simulink model "Approx_Multiplier_M2_AMA2_NAB12"  (R2021a)
settings: Solver=VariableStepAuto  StartTime=0.0  StopTime=0.01  RelTol=1e-3
(part 1 of 2)
settings Model: SimulationMode=accelerator  Creator=PC  LastModifiedBy=PC
settings DataIOCC: SaveOutput=off  SignalLogging=off  DSMLogging=off  SaveTime=off

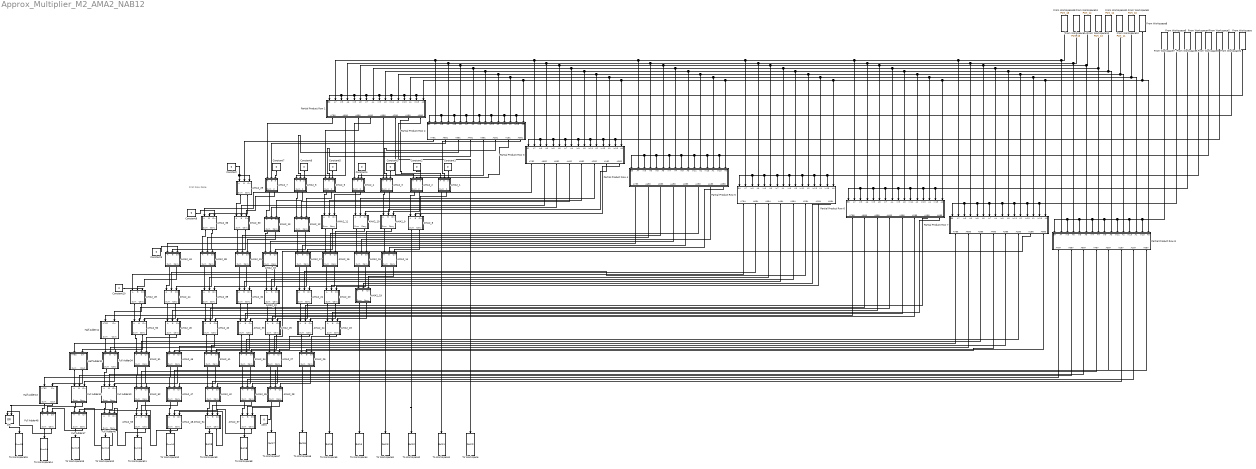
== system Approx_Multiplier_M2_AMA2_NAB12 ==
  note: First Row Done
  AMA2_1 : Subsystem
  AMA2_10 : Subsystem
  AMA2_11 : Subsystem
  AMA2_12 : Subsystem
  AMA2_13 : Subsystem
  AMA2_14 : Subsystem
  AMA2_15 : Subsystem
  AMA2_16 : Subsystem
  AMA2_17 : Subsystem
  AMA2_18 : Subsystem
  AMA2_19 : Subsystem
  AMA2_2 : Subsystem
  AMA2_20 : Subsystem
  AMA2_21 : Subsystem
  AMA2_22 : Subsystem
  AMA2_23 : Subsystem
  AMA2_24 : Subsystem
  AMA2_25 : Subsystem
  AMA2_26 : Subsystem
  AMA2_27 : Subsystem
  AMA2_28 : Subsystem
  AMA2_29 : Subsystem
  AMA2_3 : Subsystem
  AMA2_30 : Subsystem
  AMA2_31 : Subsystem
  AMA2_32 : Subsystem
  AMA2_33 : Subsystem
  AMA2_34 : Subsystem
  AMA2_35 : Subsystem
  AMA2_36 : Subsystem
  AMA2_37 : Subsystem
  AMA2_38 : Subsystem
  AMA2_39 : Subsystem
  AMA2_4 : Subsystem
  AMA2_40 : Subsystem
  AMA2_41 : Subsystem
  AMA2_42 : Subsystem
  AMA2_43 : Subsystem
  AMA2_44 : Subsystem
  AMA2_45 : Subsystem
  AMA2_46 : Subsystem
  AMA2_47 : Subsystem
  AMA2_48 : Subsystem
  AMA2_49 : Subsystem
  AMA2_5 : Subsystem
  AMA2_50 : Subsystem
  AMA2_51 : Subsystem
  AMA2_52 : Subsystem
  AMA2_53 : Subsystem
  AMA2_54 : Subsystem
  AMA2_6 : Subsystem
  AMA2_7 : Subsystem
  AMA2_8 : Subsystem
  AMA2_9 : Subsystem
  Constant{,1..10} (11 alike) : Constant  Value=0
  From Workspace : FromWorkspace  VariableName=Port_1
  From Workspace1 : FromWorkspace  VariableName=Port_2
  From Workspace10 : FromWorkspace  VariableName=Port_11
  From Workspace11 : FromWorkspace  VariableName=Port_12
  From Workspace12 : FromWorkspace  VariableName=Port_13
  From Workspace13 : FromWorkspace  VariableName=Port_14
  From Workspace14 : FromWorkspace  VariableName=Port_15
  From Workspace15 : FromWorkspace  VariableName=Port_16
  From Workspace2 : FromWorkspace  VariableName=Port_3
  From Workspace3 : FromWorkspace  VariableName=Port_4
  From Workspace4 : FromWorkspace  VariableName=Port_5
  From Workspace5 : FromWorkspace  VariableName=Port_6
  From Workspace6 : FromWorkspace  VariableName=Port_7
  From Workspace7 : FromWorkspace  VariableName=Port_8
  From Workspace8 : FromWorkspace  VariableName=Port_9
  From Workspace9 : FromWorkspace  VariableName=Port_10
  Full Adder34 : Subsystem
  Full Adder40 : Subsystem
  Full Adder41 : Subsystem
  Full Adder46 : Subsystem
  Full Adder47 : Subsystem
  Full Adder48 : Subsystem
  Half Adder11 : Subsystem
  Half Adder12 : Subsystem
  Half Adder13 : Subsystem
  OR : Logic  Operator=OR  IconShape=distinctive  AllPortsSameDT=off  OutDataTypeStr=boolean
  Partial Product Row 1 : Subsystem
  Partial Product Row 2 : Subsystem
  Partial Product Row 3 : Subsystem
  Partial Product Row 4 : Subsystem
  Partial Product Row 5 : Subsystem
  Partial Product Row 6 : Subsystem
  Partial Product Row 7 : Subsystem
  Partial Product Row 8 : Subsystem
  To Workspace : ToWorkspace  VariableName=Sum0  SampleTime=0.01
      settings: Save2DSignal=2-D array (concatenate along first dimension)
  To Workspace1 : ToWorkspace  VariableName=Sum1  SampleTime=0.01
      settings: Save2DSignal=2-D array (concatenate along first dimension)
  To Workspace10 : ToWorkspace  VariableName=Sum10  SampleTime=0.01
      settings: Save2DSignal=2-D array (concatenate along first dimension)
  To Workspace11 : ToWorkspace  VariableName=Sum11  SampleTime=0.01
      settings: Save2DSignal=2-D array (concatenate along first dimension)
  To Workspace12 : ToWorkspace  VariableName=Sum12  SampleTime=0.01
      settings: Save2DSignal=2-D array (concatenate along first dimension)
  To Workspace13 : ToWorkspace  VariableName=Sum13  SampleTime=0.01
      settings: Save2DSignal=2-D array (concatenate along first dimension)
  To Workspace14 : ToWorkspace  VariableName=Sum14  SampleTime=0.01
      settings: Save2DSignal=2-D array (concatenate along first dimension)
  To Workspace15 : ToWorkspace  VariableName=Sum15  SampleTime=0.01
      settings: Save2DSignal=2-D array (concatenate along first dimension)
  To Workspace2 : ToWorkspace  VariableName=Sum2  SampleTime=0.01
      settings: Save2DSignal=2-D array (concatenate along first dimension)
  To Workspace3 : ToWorkspace  VariableName=Sum3  SampleTime=0.01
      settings: Save2DSignal=2-D array (concatenate along first dimension)
  To Workspace4 : ToWorkspace  VariableName=Sum4  SampleTime=0.01
      settings: Save2DSignal=2-D array (concatenate along first dimension)
  To Workspace5 : ToWorkspace  VariableName=Sum5  SampleTime=0.01
      settings: Save2DSignal=2-D array (concatenate along first dimension)
  To Workspace6 : ToWorkspace  VariableName=Sum6  SampleTime=0.01
      settings: Save2DSignal=2-D array (concatenate along first dimension)
  To Workspace7 : ToWorkspace  VariableName=Sum7  SampleTime=0.01
      settings: Save2DSignal=2-D array (concatenate along first dimension)
  To Workspace8 : ToWorkspace  VariableName=Sum8  SampleTime=0.01
      settings: Save2DSignal=2-D array (concatenate along first dimension)
  To Workspace9 : ToWorkspace  VariableName=Sum9  SampleTime=0.01
      settings: Save2DSignal=2-D array (concatenate along first dimension)
  Zero : Constant  Value=0  OutDataTypeStr=Inherit: Inherit via back propagation
  wires:
  Partial Product Row 5/7(A1B4) -> AMA2_20/2(B)
  AMA2_9/2(Carry) -> AMA2_15/3(Cin)
  Partial Product Row 8/7(A1B7) -> AMA2_35/2(B)
  Full Adder48/1(Sum) -> To Workspace14/1
  Partial Product Row 4/7(A1B3) -> AMA2_15/2(B)
  Half Adder11/2(Cout) -> Half Adder12/2(Cin)
  AMA2_8/2(Carry) -> AMA2_14/3(Cin)
  Partial Product Row 6/8(A0B5) -> AMA2_23/2(B)
  AMA2_10/1(Sum) -> AMA2_15/1(A)
  From Workspace14/1 -> Partial Product Row 8/4(A6), Partial Product Row 7/4(A6), Partial Product Row 6/4(A6), Partial Product Row 5/4(A6), Partial Product Row 4/4(A6), Partial Product Row 3/4(A6), Partial Product Row 1/4(A6), Partial Product Row 2/4(A6)
  AMA2_12/1(Sum) -> AMA2_17/1(A)
  AMA2_43/2(Carry) -> AMA2_49/2(B)
  AMA2_24/2(Carry) -> AMA2_27/3(Cin)
  Partial Product Row 7/2(A6B6) -> Full Adder34/2(B)
  Partial Product Row 1/6(A2B0) -> AMA2_2/1(A)
  Partial Product Row 2/5(A3B1) -> AMA2_4/2(B)
  Constant7/1 -> AMA2_7/3(Cin)
  AMA2_17/2(Carry) -> AMA2_22/3(Cin)
  Constant2/1 -> AMA2_2/3(Cin)
  AMA2_49/2(Carry) -> Half Adder11/2(Cin)
  AMA2_3/2(Carry) -> AMA2_10/3(Cin)
  From Workspace13/1 -> Partial Product Row 8/6(A5), Partial Product Row 6/6(A5), Partial Product Row 3/6(A5), Partial Product Row 1/6(A5), Partial Product Row 2/6(A5), Partial Product Row 4/6(A5), Partial Product Row 5/6(A5), Partial Product Row 7/6(A5)
  AMA2_12/2(Carry) -> AMA2_18/3(Cin)
  AMA2_45/2(Carry) -> AMA2_51/3(Cin)
  From Workspace8/1 -> Partial Product Row 8/16(A0), Partial Product Row 7/16(A0), Partial Product Row 6/16(A0), Partial Product Row 4/16(A0), Partial Product Row 3/16(A0), Partial Product Row 1/16(A0), Partial Product Row 2/16(A0), Partial Product Row 5/16(A0)
  Partial Product Row 1/5(A3B0) -> AMA2_3/1(A)
  Full Adder34/2(Carry) -> Full Adder41/3(Cin)
  AMA2_27/2(Carry) -> AMA2_35/3(Cin)
  AMA2_54/1(Sum) -> To Workspace9/1
  Partial Product Row 3/4(A4B2) -> AMA2_12/2(B)
  AMA2_5/2(Carry) -> AMA2_12/3(Cin)
  AMA2_6/1(Sum) -> AMA2_12/1(A)
  AMA2_13/1(Sum) -> AMA2_18/1(A)
  AMA2_2/1(Sum) -> AMA2_8/1(A)
  AMA2_11/2(Carry) -> AMA2_17/3(Cin)
  AMA2_53/1(Sum) -> To Workspace11/1
  Full Adder46/1(Sum) -> To Workspace12/1
  AMA2_34/1(Sum) -> AMA2_35/1(A)
  Partial Product Row 2/8(A0B1) -> AMA2_1/2(B)
  AMA2_8/1(Sum) -> To Workspace2/1
  Partial Product Row 3/2(A6B2) -> AMA2_30/2(B)
  AMA2_2/2(Carry) -> AMA2_9/3(Cin)
  AMA2_40/2(Carry) -> AMA2_46/3(Cin)
  AMA2_37/1(Sum) -> To Workspace8/1
  AMA2_25/1(Sum) -> AMA2_27/1(A)
  Half Adder13/1(Sum) -> Full Adder48/1(A)
  Constant3/1 -> AMA2_3/3(Cin)
  Partial Product Row 7/6(A2B6) -> AMA2_34/2(B)
  Constant4/1 -> AMA2_4/3(Cin)
  AMA2_33/1(Sum) -> AMA2_34/1(A)
  Partial Product Row 4/5(A3B3) -> AMA2_17/2(B)
  AMA2_41/2(Carry) -> AMA2_47/3(Cin)
  AMA2_18/2(Carry) -> AMA2_32/3(Cin)
  AMA2_18/1(Sum) -> AMA2_22/1(A)
  Partial Product Row 3/8(A0B2) -> AMA2_8/2(B)
  Partial Product Row 2/4(A4B1) -> AMA2_5/2(B)
  Full Adder47/2(Carry) -> Full Adder48/3(Cin)
  Partial Product Row 2/3(A5B1) -> AMA2_6/2(B)
  AMA2_53/2(Carry) -> Full Adder46/3(Cin)
  Partial Product Row 6/7(A1B5) -> AMA2_24/2(B)
  From Workspace/1 -> Partial Product Row 1/3(In3), Partial Product Row 1/1(B0), Partial Product Row 1/5(In5), Partial Product Row 1/7(In7), Partial Product Row 1/9(In9), Partial Product Row 1/11(In11), Partial Product Row 1/13(In13), Partial Product Row 1/15(In15)
  AMA2_13/2(Carry) -> AMA2_31/3(Cin)
  Partial Product Row 6/4(A4B5) -> AMA2_40/2(B)
  From Workspace12/1 -> Partial Product Row 8/8(A4), Partial Product Row 6/8(A4), Partial Product Row 4/8(A4), Partial Product Row 3/8(A4), Partial Product Row 1/8(A4), Partial Product Row 2/8(A4), Partial Product Row 5/8(A4), Partial Product Row 7/8(A4)
  AMA2_37/2(Carry) -> AMA2_54/3(Cin)
  AMA2_43/1(Sum) -> AMA2_44/1(A)
  Partial Product Row 1/7(A1B0) -> AMA2_1/1(A)
  Partial Product Row 5/6(A2B4) -> AMA2_21/2(B)
  AMA2_14/1(Sum) -> To Workspace3/1
  Partial Product Row 8/8(A0B7) -> AMA2_28/2(B)
  From Workspace5/1 -> Partial Product Row 6/7(In7), Partial Product Row 6/5(In5), Partial Product Row 6/1(B5), Partial Product Row 6/3(In3), Partial Product Row 6/9(In9), Partial Product Row 6/11(In11), Partial Product Row 6/13(In13), Partial Product Row 6/15(In15)
  Partial Product Row 1/2(A6B0) -> AMA2_6/1(A)
  AMA2_44/1(Sum) -> AMA2_45/1(A)
  AMA2_45/1(Sum) -> AMA2_46/1(A)
  AMA2_19/2(Carry) -> AMA2_23/3(Cin)
  AMA2_35/1(Sum) -> AMA2_37/1(A)
  AMA2_22/1(Sum) -> AMA2_25/1(A)
  AMA2_51/2(Carry) -> Full Adder40/3(Cin)
  AMA2_54/2(Carry) -> AMA2_48/3(Cin)
  AMA2_23/1(Sum) -> To Workspace5/1
  AMA2_48/2(Carry) -> AMA2_53/3(Cin)
  AMA2_30/2(Carry) -> AMA2_38/3(Cin)
  Partial Product Row 5/1(A7B4) -> AMA2_49/1(A)
  Constant/1 -> AMA2_29/3(Cin), AMA2_29/1(A)
  Partial Product Row 1/1(A7B0) -> AMA2_7/1(A)
  AMA2_30/1(Sum) -> AMA2_31/1(A)
  Full Adder46/2(Carry) -> Full Adder47/3(Cin)
  AMA2_31/2(Carry) -> AMA2_39/3(Cin)
  Partial Product Row 7/4(A4B6) -> AMA2_46/2(B)
  Full Adder40/1(Sum) -> Full Adder46/1(A)
  AMA2_22/2(Carry) -> AMA2_33/3(Cin)
  Partial Product Row 4/3(A5B3) -> AMA2_31/2(B)
  AMA2_20/1(Sum) -> AMA2_23/1(A)
  AMA2_42/1(Sum) -> AMA2_54/1(A)
  AMA2_15/2(Carry) -> AMA2_20/3(Cin)
  AMA2_49/1(Sum) -> AMA2_50/1(A)
  From Workspace4/1 -> Partial Product Row 5/15(In15), Partial Product Row 5/13(In13), Partial Product Row 5/11(In11), Partial Product Row 5/7(In7), Partial Product Row 5/5(In5), Partial Product Row 5/1(B4), Partial Product Row 5/3(In3), Partial Product Row 5/9(In9)
  AMA2_7/2(Carry) -> AMA2_30/3(Cin)
  From Workspace7/1 -> Partial Product Row 8/11(In11), Partial Product Row 8/9(In9), Partial Product Row 8/7(In7), Partial Product Row 8/5(In5), Partial Product Row 8/3(In3), Partial Product Row 8/1(B7), Partial Product Row 8/13(In13), Partial Product Row 8/15(In15)
  AMA2_52/1(Sum) -> AMA2_53/1(A)
  AMA2_40/1(Sum) -> AMA2_41/1(A)
  AMA2_46/1(Sum) -> AMA2_47/1(A)
  AMA2_31/1(Sum) -> AMA2_32/1(A)
  Partial Product Row 5/5(A3B4) -> AMA2_22/2(B)
  AMA2_51/1(Sum) -> AMA2_52/1(A)
  Partial Product Row 7/7(A1B6) -> AMA2_27/2(B)
  Partial Product Row 7/1(A7B6) -> Half Adder12/1(A7B2)
  AMA2_29/2(Carry) -> AMA2_36/2(B)
  AMA2_41/1(Sum) -> AMA2_42/1(A)
  AMA2_9/1(Sum) -> AMA2_14/1(A)
  AMA2_38/2(Carry) -> AMA2_44/3(Cin)
  AMA2_32/1(Sum) -> AMA2_33/1(A)
  Partial Product Row 3/6(A2B2) -> AMA2_10/2(B)
  Partial Product Row 8/1(A7B7) -> Half Adder13/1(A7B2)
  Constant1/1 -> AMA2_1/3(Cin)
  Partial Product Row 7/3(A5B6) -> AMA2_51/2(B)
  Partial Product Row 5/3(A5B4) -> AMA2_39/2(B)
  AMA2_46/2(Carry) -> AMA2_52/3(Cin)
  AMA2_29/1(Sum) -> AMA2_30/1(A)
  From Workspace6/1 -> Partial Product Row 7/13(In13), Partial Product Row 7/7(In7), Partial Product Row 7/5(In5), Partial Product Row 7/1(B6), Partial Product Row 7/3(In3), Partial Product Row 7/9(In9), Partial Product Row 7/11(In11), Partial Product Row 7/15(In15)
  Partial Product Row 2/1(A7B1) -> AMA2_29/2(B)
  From Workspace3/1 -> Partial Product Row 4/13(In13), Partial Product Row 4/11(In11), Partial Product Row 4/9(In9), Partial Product Row 4/5(In5), Partial Product Row 4/3(In3), Partial Product Row 4/1(B3), Partial Product Row 4/7(In7), Partial Product Row 4/15(In15)
  From Workspace9/1 -> Partial Product Row 8/14(A1), Partial Product Row 7/14(A1), Partial Product Row 4/14(A1), Partial Product Row 1/14(A1), Partial Product Row 2/14(A1), Partial Product Row 3/14(A1), Partial Product Row 5/14(A1), Partial Product Row 6/14(A1)
  Half Adder11/1(Sum) -> Full Adder34/1(A)
  AMA2_25/2(Carry) -> AMA2_34/3(Cin)
  AMA2_3/1(Sum) -> AMA2_9/1(A)
  AMA2_39/1(Sum) -> AMA2_40/1(A)
  Partial Product Row 7/5(A3B6) -> AMA2_41/2(B)
  Half Adder12/2(Cout) -> Half Adder13/2(Cin)
  AMA2_1/1(Sum) -> To Workspace1/1
  Partial Product Row 4/2(A6B3) -> AMA2_38/2(B)
  Partial Product Row 5/8(A0B4) -> AMA2_19/2(B)
  AMA2_10/2(Carry) -> AMA2_16/3(Cin)
  AMA2_4/2(Carry) -> AMA2_11/3(Cin)
  AMA2_17/1(Sum) -> AMA2_21/1(A)
  Partial Product Row 1/3(A5B0) -> AMA2_5/1(A)
  From Workspace15/1 -> Partial Product Row 7/2(A7), Partial Product Row 5/2(A7), Partial Product Row 3/2(A7), Partial Product Row 1/2(A7), Partial Product Row 2/2(A7), Partial Product Row 4/2(A7), Partial Product Row 6/2(A7), Partial Product Row 8/2(A7)
  AMA2_11/1(Sum) -> AMA2_16/1(A)
  Partial Product Row 6/5(A3B5) -> AMA2_33/2(B)
  Partial Product Row 2/6(A2B1) -> AMA2_3/2(B)
  AMA2_26/2(Carry) -> AMA2_28/3(Cin)
  AMA2_36/1(Sum) -> AMA2_38/1(A)
  Partial Product Row 8/5(A3B7) -> AMA2_47/2(B)
  Full Adder34/1(Sum) -> Full Adder40/1(A)
  Partial Product Row 5/2(A6B4) -> AMA2_44/2(B)
  Partial Product Row 3/3(A5B2) -> AMA2_13/2(B)
  From Workspace11/1 -> Partial Product Row 8/10(A3), Partial Product Row 6/10(A3), Partial Product Row 4/10(A3), Partial Product Row 3/10(A3), Partial Product Row 1/10(A3), Partial Product Row 2/10(A3), Partial Product Row 5/10(A3), Partial Product Row 7/10(A3)
  AMA2_50/2(Carry) -> Full Adder34/3(Cin)
  Partial Product Row 6/3(A5B5) -> AMA2_45/2(B)
  AMA2_28/1(Sum) -> To Workspace7/1
  AMA2_16/1(Sum) -> AMA2_20/1(A)
  Partial Product Row 6/2(A6B5) -> AMA2_50/2(B)
  From Workspace1/1 -> Partial Product Row 2/15(In15), Partial Product Row 2/5(In5), Partial Product Row 2/3(In3), Partial Product Row 2/1(B1), Partial Product Row 2/7(In7), Partial Product Row 2/9(In9), Partial Product Row 2/11(In11), Partial Product Row 2/13(In13)
  AMA2_26/1(Sum) -> To Workspace6/1
  From Workspace10/1 -> Partial Product Row 8/12(A2), Partial Product Row 7/12(A2), Partial Product Row 5/12(A2), Partial Product Row 4/12(A2), Partial Product Row 3/12(A2), Partial Product Row 1/12(A2), Partial Product Row 2/12(A2), Partial Product Row 6/12(A2)
  Partial Product Row 8/2(A6B7) -> Full Adder41/2(B)
  Constant5/1 -> AMA2_5/3(Cin)
  AMA2_21/2(Carry) -> AMA2_25/3(Cin)
  Partial Product Row 6/1(A7B5) -> Half Adder11/1(A7B2)
  From Workspace2/1 -> Partial Product Row 3/13(In13), Partial Product Row 3/7(In7), Partial Product Row 3/5(In5), Partial Product Row 3/3(In3), Partial Product Row 3/1(B2), Partial Product Row 3/9(In9), Partial Product Row 3/11(In11), Partial Product Row 3/15(In15)
  AMA2_48/1(Sum) -> To Workspace10/1
  AMA2_15/1(Sum) -> AMA2_19/1(A)
  AMA2_20/2(Carry) -> AMA2_24/3(Cin)
  AMA2_27/1(Sum) -> AMA2_28/1(A)
  AMA2_19/1(Sum) -> To Workspace4/1
  Partial Product Row 2/2(A6B1) -> AMA2_7/2(B)
  AMA2_14/2(Carry) -> AMA2_19/3(Cin)
  Partial Product Row 4/1(A7B3) -> AMA2_43/1(A)
  Partial Product Row 3/5(A3B2) -> AMA2_11/2(B)
  AMA2_47/1(Sum) -> AMA2_48/1(A)
  Partial Product Row 3/1(A7B2) -> AMA2_36/1(A)
  Full Adder41/1(Sum) -> Full Adder47/1(A)
  AMA2_38/1(Sum) -> AMA2_39/1(A)
  AMA2_36/2(Carry) -> AMA2_43/2(B)
  AMA2_39/2(Carry) -> AMA2_45/3(Cin)
  Partial Product Row 3/7(A1B2) -> AMA2_9/2(B)
  AMA2_32/2(Carry) -> AMA2_40/3(Cin)
  Partial Product Row 8/6(A2B7) -> AMA2_42/2(B)
  AMA2_23/2(Carry) -> AMA2_26/3(Cin)
  AMA2_5/1(Sum) -> AMA2_11/1(A)
  Partial Product Row 8/3(A5B7) -> Full Adder40/2(B)
  AMA2_6/2(Carry) -> AMA2_13/3(Cin)
  AMA2_16/2(Carry) -> AMA2_21/3(Cin)
  AMA2_7/1(Sum) -> AMA2_13/1(A)
  Partial Product Row 8/4(A4B7) -> AMA2_52/2(B)
  Full Adder47/1(Sum) -> To Workspace13/1
  AMA2_21/1(Sum) -> AMA2_24/1(A)
  AMA2_4/1(Sum) -> AMA2_10/1(A)
  AMA2_33/2(Carry) -> AMA2_41/3(Cin)
  Partial Product Row 4/6(A2B3) -> AMA2_16/2(B)
  Half Adder12/1(Sum) -> Full Adder41/1(A)
  AMA2_44/2(Carry) -> AMA2_50/3(Cin)
  Partial Product Row 6/6(A2B5) -> AMA2_25/2(B)
  Partial Product Row 4/4(A4B3) -> AMA2_18/2(B)
  AMA2_1/2(Carry) -> AMA2_8/3(Cin)
  Partial Product Row 1/4(A4B0) -> AMA2_4/1(A)
  AMA2_34/2(Carry) -> AMA2_42/3(Cin)
  AMA2_24/1(Sum) -> AMA2_26/1(A)
  Constant6/1 -> AMA2_6/3(Cin)
  Partial Product Row 5/4(A4B4) -> AMA2_32/2(B)
  Partial Product Row 4/8(A0B3) -> AMA2_14/2(B)
  Partial Product Row 2/7(A1B1) -> AMA2_2/2(B)
  AMA2_50/1(Sum) -> AMA2_51/1(A)
  Partial Product Row 7/8(A0B6) -> AMA2_26/2(B)
  Partial Product Row 1/8(A0B0) -> To Workspace/1
  Half Adder13/2(Cout) -> OR/2
  Full Adder48/2(Carry) -> OR/1
  OR/1 -> To Workspace15/1
  Full Adder41/2(Carry) -> Full Adder48/2(B)
  Full Adder40/2(Carry) -> Full Adder47/2(B)
  AMA2_52/2(Carry) -> Full Adder46/2(B)
  AMA2_47/2(Carry) -> AMA2_53/2(B)
  AMA2_42/2(Carry) -> AMA2_48/2(B)
  AMA2_35/2(Carry) -> AMA2_54/2(B)
  AMA2_28/2(Carry) -> AMA2_37/2(B)
  Zero/1 -> AMA2_37/3(Cin)
  Constant8/1 -> AMA2_36/3(Cin)
  Constant9/1 -> AMA2_43/3(Cin)
  Constant10/1 -> AMA2_49/3(Cin)

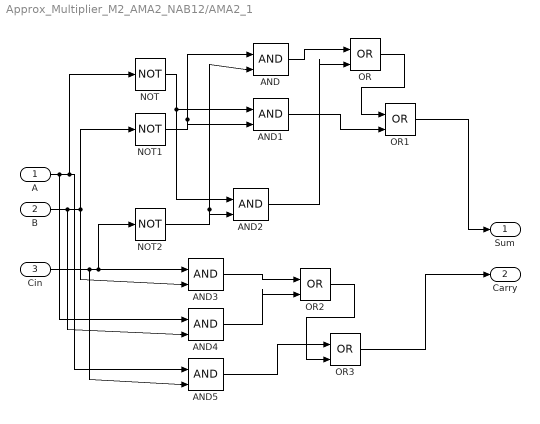
== system Approx_Multiplier_M2_AMA2_NAB12/AMA2_1 ==
  A : Inport
  B : Inport  Port=2
  Cin : Inport  Port=3
  AND{,1..5} (6 alike) : Logic  IconShape=distinctive  AllPortsSameDT=off  OutDataTypeStr=boolean
  NOT : Logic  Operator=NOT  IconShape=distinctive  AllPortsSameDT=off  OutDataTypeStr=boolean
  NOT1 : Logic  Operator=NOT  IconShape=distinctive  AllPortsSameDT=off  OutDataTypeStr=boolean
  NOT2 : Logic  Operator=NOT  IconShape=distinctive  AllPortsSameDT=off  OutDataTypeStr=boolean
  OR{,1..3} (4 alike) : Logic  Operator=OR  IconShape=distinctive  AllPortsSameDT=off  OutDataTypeStr=boolean
  Sum : Outport
  Carry : Outport  Port=2
  wires:
  A/1 -> AND4/1, AND5/1, NOT/1
  B/1 -> AND4/2, AND3/2, NOT1/1
  Cin/1 -> AND5/2, AND3/1, NOT2/1
  NOT2/1 -> AND2/2, AND/2
  NOT1/1 -> AND1/2, AND/1
  NOT/1 -> AND2/1, AND1/1
  AND2/1 -> OR/2
  AND/1 -> OR/1
  OR/1 -> OR1/1
  AND1/1 -> OR1/2
  OR1/1 -> Sum/1
  AND3/1 -> OR2/1
  AND4/1 -> OR2/2
  AND5/1 -> OR3/1
  OR2/1 -> OR3/2
  OR3/1 -> Carry/1

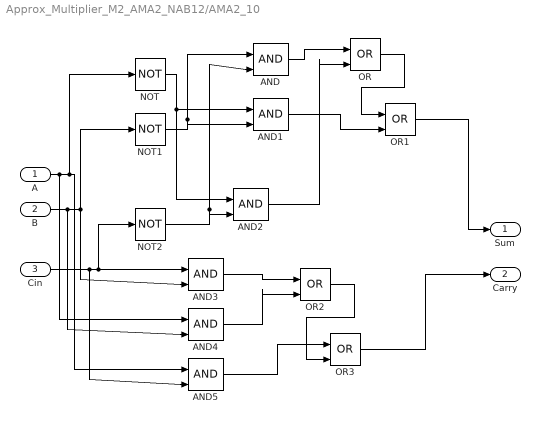
== system Approx_Multiplier_M2_AMA2_NAB12/AMA2_10 ==
  A : Inport
  B : Inport  Port=2
  Cin : Inport  Port=3
  AND{,1..5} (6 alike) : Logic  IconShape=distinctive  AllPortsSameDT=off  OutDataTypeStr=boolean
  NOT : Logic  Operator=NOT  IconShape=distinctive  AllPortsSameDT=off  OutDataTypeStr=boolean
  NOT1 : Logic  Operator=NOT  IconShape=distinctive  AllPortsSameDT=off  OutDataTypeStr=boolean
  NOT2 : Logic  Operator=NOT  IconShape=distinctive  AllPortsSameDT=off  OutDataTypeStr=boolean
  OR{,1..3} (4 alike) : Logic  Operator=OR  IconShape=distinctive  AllPortsSameDT=off  OutDataTypeStr=boolean
  Sum : Outport
  Carry : Outport  Port=2
  wires:
  A/1 -> AND4/1, AND5/1, NOT/1
  B/1 -> AND4/2, AND3/2, NOT1/1
  Cin/1 -> AND5/2, AND3/1, NOT2/1
  NOT2/1 -> AND2/2, AND/2
  NOT1/1 -> AND1/2, AND/1
  NOT/1 -> AND2/1, AND1/1
  AND2/1 -> OR/2
  AND/1 -> OR/1
  OR/1 -> OR1/1
  AND1/1 -> OR1/2
  OR1/1 -> Sum/1
  AND3/1 -> OR2/1
  AND4/1 -> OR2/2
  AND5/1 -> OR3/1
  OR2/1 -> OR3/2
  OR3/1 -> Carry/1

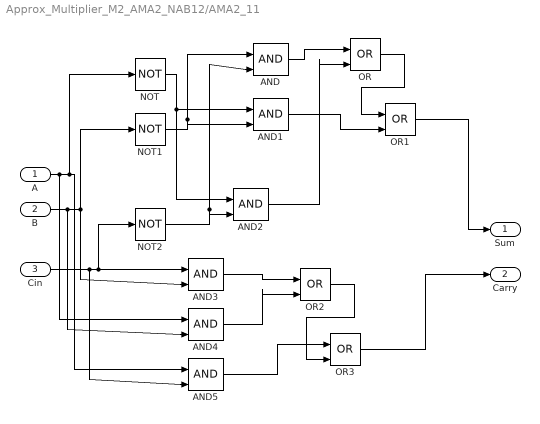
== system Approx_Multiplier_M2_AMA2_NAB12/AMA2_11 ==
  A : Inport
  B : Inport  Port=2
  Cin : Inport  Port=3
  AND{,1..5} (6 alike) : Logic  IconShape=distinctive  AllPortsSameDT=off  OutDataTypeStr=boolean
  NOT : Logic  Operator=NOT  IconShape=distinctive  AllPortsSameDT=off  OutDataTypeStr=boolean
  NOT1 : Logic  Operator=NOT  IconShape=distinctive  AllPortsSameDT=off  OutDataTypeStr=boolean
  NOT2 : Logic  Operator=NOT  IconShape=distinctive  AllPortsSameDT=off  OutDataTypeStr=boolean
  OR{,1..3} (4 alike) : Logic  Operator=OR  IconShape=distinctive  AllPortsSameDT=off  OutDataTypeStr=boolean
  Sum : Outport
  Carry : Outport  Port=2
  wires:
  A/1 -> AND4/1, AND5/1, NOT/1
  B/1 -> AND4/2, AND3/2, NOT1/1
  Cin/1 -> AND5/2, AND3/1, NOT2/1
  NOT2/1 -> AND2/2, AND/2
  NOT1/1 -> AND1/2, AND/1
  NOT/1 -> AND2/1, AND1/1
  AND2/1 -> OR/2
  AND/1 -> OR/1
  OR/1 -> OR1/1
  AND1/1 -> OR1/2
  OR1/1 -> Sum/1
  AND3/1 -> OR2/1
  AND4/1 -> OR2/2
  AND5/1 -> OR3/1
  OR2/1 -> OR3/2
  OR3/1 -> Carry/1

== system Approx_Multiplier_M2_AMA2_NAB12/AMA2_12 ==
  A : Inport
  B : Inport  Port=2
  Cin : Inport  Port=3
  AND{,1..5} (6 alike) : Logic  IconShape=distinctive  AllPortsSameDT=off  OutDataTypeStr=boolean
  NOT : Logic  Operator=NOT  IconShape=distinctive  AllPortsSameDT=off  OutDataTypeStr=boolean
  NOT1 : Logic  Operator=NOT  IconShape=distinctive  AllPortsSameDT=off  OutDataTypeStr=boolean
  NOT2 : Logic  Operator=NOT  IconShape=distinctive  AllPortsSameDT=off  OutDataTypeStr=boolean
  OR{,1..3} (4 alike) : Logic  Operator=OR  IconShape=distinctive  AllPortsSameDT=off  OutDataTypeStr=boolean
  Sum : Outport
  Carry : Outport  Port=2
  wires:
  A/1 -> AND4/1, AND5/1, NOT/1
  B/1 -> AND4/2, AND3/2, NOT1/1
  Cin/1 -> AND5/2, AND3/1, NOT2/1
  NOT2/1 -> AND2/2, AND/2
  NOT1/1 -> AND1/2, AND/1
  NOT/1 -> AND2/1, AND1/1
  AND2/1 -> OR/2
  AND/1 -> OR/1
  OR/1 -> OR1/1
  AND1/1 -> OR1/2
  OR1/1 -> Sum/1
  AND3/1 -> OR2/1
  AND4/1 -> OR2/2
  AND5/1 -> OR3/1
  OR2/1 -> OR3/2
  OR3/1 -> Carry/1

== system Approx_Multiplier_M2_AMA2_NAB12/AMA2_13 ==
  A : Inport
  B : Inport  Port=2
  Cin : Inport  Port=3
  AND{,1..5} (6 alike) : Logic  IconShape=distinctive  AllPortsSameDT=off  OutDataTypeStr=boolean
  NOT : Logic  Operator=NOT  IconShape=distinctive  AllPortsSameDT=off  OutDataTypeStr=boolean
  NOT1 : Logic  Operator=NOT  IconShape=distinctive  AllPortsSameDT=off  OutDataTypeStr=boolean
  NOT2 : Logic  Operator=NOT  IconShape=distinctive  AllPortsSameDT=off  OutDataTypeStr=boolean
  OR{,1..3} (4 alike) : Logic  Operator=OR  IconShape=distinctive  AllPortsSameDT=off  OutDataTypeStr=boolean
  Sum : Outport
  Carry : Outport  Port=2
  wires:
  A/1 -> AND4/1, AND5/1, NOT/1
  B/1 -> AND4/2, AND3/2, NOT1/1
  Cin/1 -> AND5/2, AND3/1, NOT2/1
  NOT2/1 -> AND2/2, AND/2
  NOT1/1 -> AND1/2, AND/1
  NOT/1 -> AND2/1, AND1/1
  AND2/1 -> OR/2
  AND/1 -> OR/1
  OR/1 -> OR1/1
  AND1/1 -> OR1/2
  OR1/1 -> Sum/1
  AND3/1 -> OR2/1
  AND4/1 -> OR2/2
  AND5/1 -> OR3/1
  OR2/1 -> OR3/2
  OR3/1 -> Carry/1

== system Approx_Multiplier_M2_AMA2_NAB12/AMA2_14 ==
  A : Inport
  B : Inport  Port=2
  Cin : Inport  Port=3
  AND{,1..5} (6 alike) : Logic  IconShape=distinctive  AllPortsSameDT=off  OutDataTypeStr=boolean
  NOT : Logic  Operator=NOT  IconShape=distinctive  AllPortsSameDT=off  OutDataTypeStr=boolean
  NOT1 : Logic  Operator=NOT  IconShape=distinctive  AllPortsSameDT=off  OutDataTypeStr=boolean
  NOT2 : Logic  Operator=NOT  IconShape=distinctive  AllPortsSameDT=off  OutDataTypeStr=boolean
  OR{,1..3} (4 alike) : Logic  Operator=OR  IconShape=distinctive  AllPortsSameDT=off  OutDataTypeStr=boolean
  Sum : Outport
  Carry : Outport  Port=2
  wires:
  A/1 -> AND4/1, AND5/1, NOT/1
  B/1 -> AND4/2, AND3/2, NOT1/1
  Cin/1 -> AND5/2, AND3/1, NOT2/1
  NOT2/1 -> AND2/2, AND/2
  NOT1/1 -> AND1/2, AND/1
  NOT/1 -> AND2/1, AND1/1
  AND2/1 -> OR/2
  AND/1 -> OR/1
  OR/1 -> OR1/1
  AND1/1 -> OR1/2
  OR1/1 -> Sum/1
  AND3/1 -> OR2/1
  AND4/1 -> OR2/2
  AND5/1 -> OR3/1
  OR2/1 -> OR3/2
  OR3/1 -> Carry/1

== system Approx_Multiplier_M2_AMA2_NAB12/AMA2_15 ==
  A : Inport
  B : Inport  Port=2
  Cin : Inport  Port=3
  AND{,1..5} (6 alike) : Logic  IconShape=distinctive  AllPortsSameDT=off  OutDataTypeStr=boolean
  NOT : Logic  Operator=NOT  IconShape=distinctive  AllPortsSameDT=off  OutDataTypeStr=boolean
  NOT1 : Logic  Operator=NOT  IconShape=distinctive  AllPortsSameDT=off  OutDataTypeStr=boolean
  NOT2 : Logic  Operator=NOT  IconShape=distinctive  AllPortsSameDT=off  OutDataTypeStr=boolean
  OR{,1..3} (4 alike) : Logic  Operator=OR  IconShape=distinctive  AllPortsSameDT=off  OutDataTypeStr=boolean
  Sum : Outport
  Carry : Outport  Port=2
  wires:
  A/1 -> AND4/1, AND5/1, NOT/1
  B/1 -> AND4/2, AND3/2, NOT1/1
  Cin/1 -> AND5/2, AND3/1, NOT2/1
  NOT2/1 -> AND2/2, AND/2
  NOT1/1 -> AND1/2, AND/1
  NOT/1 -> AND2/1, AND1/1
  AND2/1 -> OR/2
  AND/1 -> OR/1
  OR/1 -> OR1/1
  AND1/1 -> OR1/2
  OR1/1 -> Sum/1
  AND3/1 -> OR2/1
  AND4/1 -> OR2/2
  AND5/1 -> OR3/1
  OR2/1 -> OR3/2
  OR3/1 -> Carry/1

== system Approx_Multiplier_M2_AMA2_NAB12/AMA2_16 ==
  A : Inport
  B : Inport  Port=2
  Cin : Inport  Port=3
  AND{,1..5} (6 alike) : Logic  IconShape=distinctive  AllPortsSameDT=off  OutDataTypeStr=boolean
  NOT : Logic  Operator=NOT  IconShape=distinctive  AllPortsSameDT=off  OutDataTypeStr=boolean
  NOT1 : Logic  Operator=NOT  IconShape=distinctive  AllPortsSameDT=off  OutDataTypeStr=boolean
  NOT2 : Logic  Operator=NOT  IconShape=distinctive  AllPortsSameDT=off  OutDataTypeStr=boolean
  OR{,1..3} (4 alike) : Logic  Operator=OR  IconShape=distinctive  AllPortsSameDT=off  OutDataTypeStr=boolean
  Sum : Outport
  Carry : Outport  Port=2
  wires:
  A/1 -> AND4/1, AND5/1, NOT/1
  B/1 -> AND4/2, AND3/2, NOT1/1
  Cin/1 -> AND5/2, AND3/1, NOT2/1
  NOT2/1 -> AND2/2, AND/2
  NOT1/1 -> AND1/2, AND/1
  NOT/1 -> AND2/1, AND1/1
  AND2/1 -> OR/2
  AND/1 -> OR/1
  OR/1 -> OR1/1
  AND1/1 -> OR1/2
  OR1/1 -> Sum/1
  AND3/1 -> OR2/1
  AND4/1 -> OR2/2
  AND5/1 -> OR3/1
  OR2/1 -> OR3/2
  OR3/1 -> Carry/1

== system Approx_Multiplier_M2_AMA2_NAB12/AMA2_17 ==
  A : Inport
  B : Inport  Port=2
  Cin : Inport  Port=3
  AND{,1..5} (6 alike) : Logic  IconShape=distinctive  AllPortsSameDT=off  OutDataTypeStr=boolean
  NOT : Logic  Operator=NOT  IconShape=distinctive  AllPortsSameDT=off  OutDataTypeStr=boolean
  NOT1 : Logic  Operator=NOT  IconShape=distinctive  AllPortsSameDT=off  OutDataTypeStr=boolean
  NOT2 : Logic  Operator=NOT  IconShape=distinctive  AllPortsSameDT=off  OutDataTypeStr=boolean
  OR{,1..3} (4 alike) : Logic  Operator=OR  IconShape=distinctive  AllPortsSameDT=off  OutDataTypeStr=boolean
  Sum : Outport
  Carry : Outport  Port=2
  wires:
  A/1 -> AND4/1, AND5/1, NOT/1
  B/1 -> AND4/2, AND3/2, NOT1/1
  Cin/1 -> AND5/2, AND3/1, NOT2/1
  NOT2/1 -> AND2/2, AND/2
  NOT1/1 -> AND1/2, AND/1
  NOT/1 -> AND2/1, AND1/1
  AND2/1 -> OR/2
  AND/1 -> OR/1
  OR/1 -> OR1/1
  AND1/1 -> OR1/2
  OR1/1 -> Sum/1
  AND3/1 -> OR2/1
  AND4/1 -> OR2/2
  AND5/1 -> OR3/1
  OR2/1 -> OR3/2
  OR3/1 -> Carry/1

== system Approx_Multiplier_M2_AMA2_NAB12/AMA2_18 ==
  A : Inport
  B : Inport  Port=2
  Cin : Inport  Port=3
  AND{,1..5} (6 alike) : Logic  IconShape=distinctive  AllPortsSameDT=off  OutDataTypeStr=boolean
  NOT : Logic  Operator=NOT  IconShape=distinctive  AllPortsSameDT=off  OutDataTypeStr=boolean
  NOT1 : Logic  Operator=NOT  IconShape=distinctive  AllPortsSameDT=off  OutDataTypeStr=boolean
  NOT2 : Logic  Operator=NOT  IconShape=distinctive  AllPortsSameDT=off  OutDataTypeStr=boolean
  OR{,1..3} (4 alike) : Logic  Operator=OR  IconShape=distinctive  AllPortsSameDT=off  OutDataTypeStr=boolean
  Sum : Outport
  Carry : Outport  Port=2
  wires:
  A/1 -> AND4/1, AND5/1, NOT/1
  B/1 -> AND4/2, AND3/2, NOT1/1
  Cin/1 -> AND5/2, AND3/1, NOT2/1
  NOT2/1 -> AND2/2, AND/2
  NOT1/1 -> AND1/2, AND/1
  NOT/1 -> AND2/1, AND1/1
  AND2/1 -> OR/2
  AND/1 -> OR/1
  OR/1 -> OR1/1
  AND1/1 -> OR1/2
  OR1/1 -> Sum/1
  AND3/1 -> OR2/1
  AND4/1 -> OR2/2
  AND5/1 -> OR3/1
  OR2/1 -> OR3/2
  OR3/1 -> Carry/1

== system Approx_Multiplier_M2_AMA2_NAB12/AMA2_19 ==
  A : Inport
  B : Inport  Port=2
  Cin : Inport  Port=3
  AND{,1..5} (6 alike) : Logic  IconShape=distinctive  AllPortsSameDT=off  OutDataTypeStr=boolean
  NOT : Logic  Operator=NOT  IconShape=distinctive  AllPortsSameDT=off  OutDataTypeStr=boolean
  NOT1 : Logic  Operator=NOT  IconShape=distinctive  AllPortsSameDT=off  OutDataTypeStr=boolean
  NOT2 : Logic  Operator=NOT  IconShape=distinctive  AllPortsSameDT=off  OutDataTypeStr=boolean
  OR{,1..3} (4 alike) : Logic  Operator=OR  IconShape=distinctive  AllPortsSameDT=off  OutDataTypeStr=boolean
  Sum : Outport
  Carry : Outport  Port=2
  wires:
  A/1 -> AND4/1, AND5/1, NOT/1
  B/1 -> AND4/2, AND3/2, NOT1/1
  Cin/1 -> AND5/2, AND3/1, NOT2/1
  NOT2/1 -> AND2/2, AND/2
  NOT1/1 -> AND1/2, AND/1
  NOT/1 -> AND2/1, AND1/1
  AND2/1 -> OR/2
  AND/1 -> OR/1
  OR/1 -> OR1/1
  AND1/1 -> OR1/2
  OR1/1 -> Sum/1
  AND3/1 -> OR2/1
  AND4/1 -> OR2/2
  AND5/1 -> OR3/1
  OR2/1 -> OR3/2
  OR3/1 -> Carry/1

== system Approx_Multiplier_M2_AMA2_NAB12/AMA2_2 ==
  A : Inport
  B : Inport  Port=2
  Cin : Inport  Port=3
  AND{,1..5} (6 alike) : Logic  IconShape=distinctive  AllPortsSameDT=off  OutDataTypeStr=boolean
  NOT : Logic  Operator=NOT  IconShape=distinctive  AllPortsSameDT=off  OutDataTypeStr=boolean
  NOT1 : Logic  Operator=NOT  IconShape=distinctive  AllPortsSameDT=off  OutDataTypeStr=boolean
  NOT2 : Logic  Operator=NOT  IconShape=distinctive  AllPortsSameDT=off  OutDataTypeStr=boolean
  OR{,1..3} (4 alike) : Logic  Operator=OR  IconShape=distinctive  AllPortsSameDT=off  OutDataTypeStr=boolean
  Sum : Outport
  Carry : Outport  Port=2
  wires:
  A/1 -> AND4/1, AND5/1, NOT/1
  B/1 -> AND4/2, AND3/2, NOT1/1
  Cin/1 -> AND5/2, AND3/1, NOT2/1
  NOT2/1 -> AND2/2, AND/2
  NOT1/1 -> AND1/2, AND/1
  NOT/1 -> AND2/1, AND1/1
  AND2/1 -> OR/2
  AND/1 -> OR/1
  OR/1 -> OR1/1
  AND1/1 -> OR1/2
  OR1/1 -> Sum/1
  AND3/1 -> OR2/1
  AND4/1 -> OR2/2
  AND5/1 -> OR3/1
  OR2/1 -> OR3/2
  OR3/1 -> Carry/1

== system Approx_Multiplier_M2_AMA2_NAB12/AMA2_20 ==
  A : Inport
  B : Inport  Port=2
  Cin : Inport  Port=3
  AND{,1..5} (6 alike) : Logic  IconShape=distinctive  AllPortsSameDT=off  OutDataTypeStr=boolean
  NOT : Logic  Operator=NOT  IconShape=distinctive  AllPortsSameDT=off  OutDataTypeStr=boolean
  NOT1 : Logic  Operator=NOT  IconShape=distinctive  AllPortsSameDT=off  OutDataTypeStr=boolean
  NOT2 : Logic  Operator=NOT  IconShape=distinctive  AllPortsSameDT=off  OutDataTypeStr=boolean
  OR{,1..3} (4 alike) : Logic  Operator=OR  IconShape=distinctive  AllPortsSameDT=off  OutDataTypeStr=boolean
  Sum : Outport
  Carry : Outport  Port=2
  wires:
  A/1 -> AND4/1, AND5/1, NOT/1
  B/1 -> AND4/2, AND3/2, NOT1/1
  Cin/1 -> AND5/2, AND3/1, NOT2/1
  NOT2/1 -> AND2/2, AND/2
  NOT1/1 -> AND1/2, AND/1
  NOT/1 -> AND2/1, AND1/1
  AND2/1 -> OR/2
  AND/1 -> OR/1
  OR/1 -> OR1/1
  AND1/1 -> OR1/2
  OR1/1 -> Sum/1
  AND3/1 -> OR2/1
  AND4/1 -> OR2/2
  AND5/1 -> OR3/1
  OR2/1 -> OR3/2
  OR3/1 -> Carry/1

== system Approx_Multiplier_M2_AMA2_NAB12/AMA2_21 ==
  A : Inport
  B : Inport  Port=2
  Cin : Inport  Port=3
  AND{,1..5} (6 alike) : Logic  IconShape=distinctive  AllPortsSameDT=off  OutDataTypeStr=boolean
  NOT : Logic  Operator=NOT  IconShape=distinctive  AllPortsSameDT=off  OutDataTypeStr=boolean
  NOT1 : Logic  Operator=NOT  IconShape=distinctive  AllPortsSameDT=off  OutDataTypeStr=boolean
  NOT2 : Logic  Operator=NOT  IconShape=distinctive  AllPortsSameDT=off  OutDataTypeStr=boolean
  OR{,1..3} (4 alike) : Logic  Operator=OR  IconShape=distinctive  AllPortsSameDT=off  OutDataTypeStr=boolean
  Sum : Outport
  Carry : Outport  Port=2
  wires:
  A/1 -> AND4/1, AND5/1, NOT/1
  B/1 -> AND4/2, AND3/2, NOT1/1
  Cin/1 -> AND5/2, AND3/1, NOT2/1
  NOT2/1 -> AND2/2, AND/2
  NOT1/1 -> AND1/2, AND/1
  NOT/1 -> AND2/1, AND1/1
  AND2/1 -> OR/2
  AND/1 -> OR/1
  OR/1 -> OR1/1
  AND1/1 -> OR1/2
  OR1/1 -> Sum/1
  AND3/1 -> OR2/1
  AND4/1 -> OR2/2
  AND5/1 -> OR3/1
  OR2/1 -> OR3/2
  OR3/1 -> Carry/1

== system Approx_Multiplier_M2_AMA2_NAB12/AMA2_22 ==
  A : Inport
  B : Inport  Port=2
  Cin : Inport  Port=3
  AND{,1..5} (6 alike) : Logic  IconShape=distinctive  AllPortsSameDT=off  OutDataTypeStr=boolean
  NOT : Logic  Operator=NOT  IconShape=distinctive  AllPortsSameDT=off  OutDataTypeStr=boolean
  NOT1 : Logic  Operator=NOT  IconShape=distinctive  AllPortsSameDT=off  OutDataTypeStr=boolean
  NOT2 : Logic  Operator=NOT  IconShape=distinctive  AllPortsSameDT=off  OutDataTypeStr=boolean
  OR{,1..3} (4 alike) : Logic  Operator=OR  IconShape=distinctive  AllPortsSameDT=off  OutDataTypeStr=boolean
  Sum : Outport
  Carry : Outport  Port=2
  wires:
  A/1 -> AND4/1, AND5/1, NOT/1
  B/1 -> AND4/2, AND3/2, NOT1/1
  Cin/1 -> AND5/2, AND3/1, NOT2/1
  NOT2/1 -> AND2/2, AND/2
  NOT1/1 -> AND1/2, AND/1
  NOT/1 -> AND2/1, AND1/1
  AND2/1 -> OR/2
  AND/1 -> OR/1
  OR/1 -> OR1/1
  AND1/1 -> OR1/2
  OR1/1 -> Sum/1
  AND3/1 -> OR2/1
  AND4/1 -> OR2/2
  AND5/1 -> OR3/1
  OR2/1 -> OR3/2
  OR3/1 -> Carry/1

== system Approx_Multiplier_M2_AMA2_NAB12/AMA2_23 ==
  A : Inport
  B : Inport  Port=2
  Cin : Inport  Port=3
  AND{,1..5} (6 alike) : Logic  IconShape=distinctive  AllPortsSameDT=off  OutDataTypeStr=boolean
  NOT : Logic  Operator=NOT  IconShape=distinctive  AllPortsSameDT=off  OutDataTypeStr=boolean
  NOT1 : Logic  Operator=NOT  IconShape=distinctive  AllPortsSameDT=off  OutDataTypeStr=boolean
  NOT2 : Logic  Operator=NOT  IconShape=distinctive  AllPortsSameDT=off  OutDataTypeStr=boolean
  OR{,1..3} (4 alike) : Logic  Operator=OR  IconShape=distinctive  AllPortsSameDT=off  OutDataTypeStr=boolean
  Sum : Outport
  Carry : Outport  Port=2
  wires:
  A/1 -> AND4/1, AND5/1, NOT/1
  B/1 -> AND4/2, AND3/2, NOT1/1
  Cin/1 -> AND5/2, AND3/1, NOT2/1
  NOT2/1 -> AND2/2, AND/2
  NOT1/1 -> AND1/2, AND/1
  NOT/1 -> AND2/1, AND1/1
  AND2/1 -> OR/2
  AND/1 -> OR/1
  OR/1 -> OR1/1
  AND1/1 -> OR1/2
  OR1/1 -> Sum/1
  AND3/1 -> OR2/1
  AND4/1 -> OR2/2
  AND5/1 -> OR3/1
  OR2/1 -> OR3/2
  OR3/1 -> Carry/1

== system Approx_Multiplier_M2_AMA2_NAB12/AMA2_24 ==
  A : Inport
  B : Inport  Port=2
  Cin : Inport  Port=3
  AND{,1..5} (6 alike) : Logic  IconShape=distinctive  AllPortsSameDT=off  OutDataTypeStr=boolean
  NOT : Logic  Operator=NOT  IconShape=distinctive  AllPortsSameDT=off  OutDataTypeStr=boolean
  NOT1 : Logic  Operator=NOT  IconShape=distinctive  AllPortsSameDT=off  OutDataTypeStr=boolean
  NOT2 : Logic  Operator=NOT  IconShape=distinctive  AllPortsSameDT=off  OutDataTypeStr=boolean
  OR{,1..3} (4 alike) : Logic  Operator=OR  IconShape=distinctive  AllPortsSameDT=off  OutDataTypeStr=boolean
  Sum : Outport
  Carry : Outport  Port=2
  wires:
  A/1 -> AND4/1, AND5/1, NOT/1
  B/1 -> AND4/2, AND3/2, NOT1/1
  Cin/1 -> AND5/2, AND3/1, NOT2/1
  NOT2/1 -> AND2/2, AND/2
  NOT1/1 -> AND1/2, AND/1
  NOT/1 -> AND2/1, AND1/1
  AND2/1 -> OR/2
  AND/1 -> OR/1
  OR/1 -> OR1/1
  AND1/1 -> OR1/2
  OR1/1 -> Sum/1
  AND3/1 -> OR2/1
  AND4/1 -> OR2/2
  AND5/1 -> OR3/1
  OR2/1 -> OR3/2
  OR3/1 -> Carry/1

== system Approx_Multiplier_M2_AMA2_NAB12/AMA2_25 ==
  A : Inport
  B : Inport  Port=2
  Cin : Inport  Port=3
  AND{,1..5} (6 alike) : Logic  IconShape=distinctive  AllPortsSameDT=off  OutDataTypeStr=boolean
  NOT : Logic  Operator=NOT  IconShape=distinctive  AllPortsSameDT=off  OutDataTypeStr=boolean
  NOT1 : Logic  Operator=NOT  IconShape=distinctive  AllPortsSameDT=off  OutDataTypeStr=boolean
  NOT2 : Logic  Operator=NOT  IconShape=distinctive  AllPortsSameDT=off  OutDataTypeStr=boolean
  OR{,1..3} (4 alike) : Logic  Operator=OR  IconShape=distinctive  AllPortsSameDT=off  OutDataTypeStr=boolean
  Sum : Outport
  Carry : Outport  Port=2
  wires:
  A/1 -> AND4/1, AND5/1, NOT/1
  B/1 -> AND4/2, AND3/2, NOT1/1
  Cin/1 -> AND5/2, AND3/1, NOT2/1
  NOT2/1 -> AND2/2, AND/2
  NOT1/1 -> AND1/2, AND/1
  NOT/1 -> AND2/1, AND1/1
  AND2/1 -> OR/2
  AND/1 -> OR/1
  OR/1 -> OR1/1
  AND1/1 -> OR1/2
  OR1/1 -> Sum/1
  AND3/1 -> OR2/1
  AND4/1 -> OR2/2
  AND5/1 -> OR3/1
  OR2/1 -> OR3/2
  OR3/1 -> Carry/1

== system Approx_Multiplier_M2_AMA2_NAB12/AMA2_26 ==
  A : Inport
  B : Inport  Port=2
  Cin : Inport  Port=3
  AND{,1..5} (6 alike) : Logic  IconShape=distinctive  AllPortsSameDT=off  OutDataTypeStr=boolean
  NOT : Logic  Operator=NOT  IconShape=distinctive  AllPortsSameDT=off  OutDataTypeStr=boolean
  NOT1 : Logic  Operator=NOT  IconShape=distinctive  AllPortsSameDT=off  OutDataTypeStr=boolean
  NOT2 : Logic  Operator=NOT  IconShape=distinctive  AllPortsSameDT=off  OutDataTypeStr=boolean
  OR{,1..3} (4 alike) : Logic  Operator=OR  IconShape=distinctive  AllPortsSameDT=off  OutDataTypeStr=boolean
  Sum : Outport
  Carry : Outport  Port=2
  wires:
  A/1 -> AND4/1, AND5/1, NOT/1
  B/1 -> AND4/2, AND3/2, NOT1/1
  Cin/1 -> AND5/2, AND3/1, NOT2/1
  NOT2/1 -> AND2/2, AND/2
  NOT1/1 -> AND1/2, AND/1
  NOT/1 -> AND2/1, AND1/1
  AND2/1 -> OR/2
  AND/1 -> OR/1
  OR/1 -> OR1/1
  AND1/1 -> OR1/2
  OR1/1 -> Sum/1
  AND3/1 -> OR2/1
  AND4/1 -> OR2/2
  AND5/1 -> OR3/1
  OR2/1 -> OR3/2
  OR3/1 -> Carry/1

== system Approx_Multiplier_M2_AMA2_NAB12/AMA2_27 ==
  A : Inport
  B : Inport  Port=2
  Cin : Inport  Port=3
  AND{,1..5} (6 alike) : Logic  IconShape=distinctive  AllPortsSameDT=off  OutDataTypeStr=boolean
  NOT : Logic  Operator=NOT  IconShape=distinctive  AllPortsSameDT=off  OutDataTypeStr=boolean
  NOT1 : Logic  Operator=NOT  IconShape=distinctive  AllPortsSameDT=off  OutDataTypeStr=boolean
  NOT2 : Logic  Operator=NOT  IconShape=distinctive  AllPortsSameDT=off  OutDataTypeStr=boolean
  OR{,1..3} (4 alike) : Logic  Operator=OR  IconShape=distinctive  AllPortsSameDT=off  OutDataTypeStr=boolean
  Sum : Outport
  Carry : Outport  Port=2
  wires:
  A/1 -> AND4/1, AND5/1, NOT/1
  B/1 -> AND4/2, AND3/2, NOT1/1
  Cin/1 -> AND5/2, AND3/1, NOT2/1
  NOT2/1 -> AND2/2, AND/2
  NOT1/1 -> AND1/2, AND/1
  NOT/1 -> AND2/1, AND1/1
  AND2/1 -> OR/2
  AND/1 -> OR/1
  OR/1 -> OR1/1
  AND1/1 -> OR1/2
  OR1/1 -> Sum/1
  AND3/1 -> OR2/1
  AND4/1 -> OR2/2
  AND5/1 -> OR3/1
  OR2/1 -> OR3/2
  OR3/1 -> Carry/1

== system Approx_Multiplier_M2_AMA2_NAB12/AMA2_28 ==
  A : Inport
  B : Inport  Port=2
  Cin : Inport  Port=3
  AND{,1..5} (6 alike) : Logic  IconShape=distinctive  AllPortsSameDT=off  OutDataTypeStr=boolean
  NOT : Logic  Operator=NOT  IconShape=distinctive  AllPortsSameDT=off  OutDataTypeStr=boolean
  NOT1 : Logic  Operator=NOT  IconShape=distinctive  AllPortsSameDT=off  OutDataTypeStr=boolean
  NOT2 : Logic  Operator=NOT  IconShape=distinctive  AllPortsSameDT=off  OutDataTypeStr=boolean
  OR{,1..3} (4 alike) : Logic  Operator=OR  IconShape=distinctive  AllPortsSameDT=off  OutDataTypeStr=boolean
  Sum : Outport
  Carry : Outport  Port=2
  wires:
  A/1 -> AND4/1, AND5/1, NOT/1
  B/1 -> AND4/2, AND3/2, NOT1/1
  Cin/1 -> AND5/2, AND3/1, NOT2/1
  NOT2/1 -> AND2/2, AND/2
  NOT1/1 -> AND1/2, AND/1
  NOT/1 -> AND2/1, AND1/1
  AND2/1 -> OR/2
  AND/1 -> OR/1
  OR/1 -> OR1/1
  AND1/1 -> OR1/2
  OR1/1 -> Sum/1
  AND3/1 -> OR2/1
  AND4/1 -> OR2/2
  AND5/1 -> OR3/1
  OR2/1 -> OR3/2
  OR3/1 -> Carry/1

== system Approx_Multiplier_M2_AMA2_NAB12/AMA2_29 ==
  A : Inport
  B : Inport  Port=2
  Cin : Inport  Port=3
  AND{,1..5} (6 alike) : Logic  IconShape=distinctive  AllPortsSameDT=off  OutDataTypeStr=boolean
  NOT : Logic  Operator=NOT  IconShape=distinctive  AllPortsSameDT=off  OutDataTypeStr=boolean
  NOT1 : Logic  Operator=NOT  IconShape=distinctive  AllPortsSameDT=off  OutDataTypeStr=boolean
  NOT2 : Logic  Operator=NOT  IconShape=distinctive  AllPortsSameDT=off  OutDataTypeStr=boolean
  OR{,1..3} (4 alike) : Logic  Operator=OR  IconShape=distinctive  AllPortsSameDT=off  OutDataTypeStr=boolean
  Sum : Outport
  Carry : Outport  Port=2
  wires:
  A/1 -> AND4/1, AND5/1, NOT/1
  B/1 -> AND4/2, AND3/2, NOT1/1
  Cin/1 -> AND5/2, AND3/1, NOT2/1
  NOT2/1 -> AND2/2, AND/2
  NOT1/1 -> AND1/2, AND/1
  NOT/1 -> AND2/1, AND1/1
  AND2/1 -> OR/2
  AND/1 -> OR/1
  OR/1 -> OR1/1
  AND1/1 -> OR1/2
  OR1/1 -> Sum/1
  AND3/1 -> OR2/1
  AND4/1 -> OR2/2
  AND5/1 -> OR3/1
  OR2/1 -> OR3/2
  OR3/1 -> Carry/1

== system Approx_Multiplier_M2_AMA2_NAB12/AMA2_3 ==
  A : Inport
  B : Inport  Port=2
  Cin : Inport  Port=3
  AND{,1..5} (6 alike) : Logic  IconShape=distinctive  AllPortsSameDT=off  OutDataTypeStr=boolean
  NOT : Logic  Operator=NOT  IconShape=distinctive  AllPortsSameDT=off  OutDataTypeStr=boolean
  NOT1 : Logic  Operator=NOT  IconShape=distinctive  AllPortsSameDT=off  OutDataTypeStr=boolean
  NOT2 : Logic  Operator=NOT  IconShape=distinctive  AllPortsSameDT=off  OutDataTypeStr=boolean
  OR{,1..3} (4 alike) : Logic  Operator=OR  IconShape=distinctive  AllPortsSameDT=off  OutDataTypeStr=boolean
  Sum : Outport
  Carry : Outport  Port=2
  wires:
  A/1 -> AND4/1, AND5/1, NOT/1
  B/1 -> AND4/2, AND3/2, NOT1/1
  Cin/1 -> AND5/2, AND3/1, NOT2/1
  NOT2/1 -> AND2/2, AND/2
  NOT1/1 -> AND1/2, AND/1
  NOT/1 -> AND2/1, AND1/1
  AND2/1 -> OR/2
  AND/1 -> OR/1
  OR/1 -> OR1/1
  AND1/1 -> OR1/2
  OR1/1 -> Sum/1
  AND3/1 -> OR2/1
  AND4/1 -> OR2/2
  AND5/1 -> OR3/1
  OR2/1 -> OR3/2
  OR3/1 -> Carry/1

== system Approx_Multiplier_M2_AMA2_NAB12/AMA2_30 ==
  A : Inport
  B : Inport  Port=2
  Cin : Inport  Port=3
  AND{,1..5} (6 alike) : Logic  IconShape=distinctive  AllPortsSameDT=off  OutDataTypeStr=boolean
  NOT : Logic  Operator=NOT  IconShape=distinctive  AllPortsSameDT=off  OutDataTypeStr=boolean
  NOT1 : Logic  Operator=NOT  IconShape=distinctive  AllPortsSameDT=off  OutDataTypeStr=boolean
  NOT2 : Logic  Operator=NOT  IconShape=distinctive  AllPortsSameDT=off  OutDataTypeStr=boolean
  OR{,1..3} (4 alike) : Logic  Operator=OR  IconShape=distinctive  AllPortsSameDT=off  OutDataTypeStr=boolean
  Sum : Outport
  Carry : Outport  Port=2
  wires:
  A/1 -> AND4/1, AND5/1, NOT/1
  B/1 -> AND4/2, AND3/2, NOT1/1
  Cin/1 -> AND5/2, AND3/1, NOT2/1
  NOT2/1 -> AND2/2, AND/2
  NOT1/1 -> AND1/2, AND/1
  NOT/1 -> AND2/1, AND1/1
  AND2/1 -> OR/2
  AND/1 -> OR/1
  OR/1 -> OR1/1
  AND1/1 -> OR1/2
  OR1/1 -> Sum/1
  AND3/1 -> OR2/1
  AND4/1 -> OR2/2
  AND5/1 -> OR3/1
  OR2/1 -> OR3/2
  OR3/1 -> Carry/1

== system Approx_Multiplier_M2_AMA2_NAB12/AMA2_31 ==
  A : Inport
  B : Inport  Port=2
  Cin : Inport  Port=3
  AND{,1..5} (6 alike) : Logic  IconShape=distinctive  AllPortsSameDT=off  OutDataTypeStr=boolean
  NOT : Logic  Operator=NOT  IconShape=distinctive  AllPortsSameDT=off  OutDataTypeStr=boolean
  NOT1 : Logic  Operator=NOT  IconShape=distinctive  AllPortsSameDT=off  OutDataTypeStr=boolean
  NOT2 : Logic  Operator=NOT  IconShape=distinctive  AllPortsSameDT=off  OutDataTypeStr=boolean
  OR{,1..3} (4 alike) : Logic  Operator=OR  IconShape=distinctive  AllPortsSameDT=off  OutDataTypeStr=boolean
  Sum : Outport
  Carry : Outport  Port=2
  wires:
  A/1 -> AND4/1, AND5/1, NOT/1
  B/1 -> AND4/2, AND3/2, NOT1/1
  Cin/1 -> AND5/2, AND3/1, NOT2/1
  NOT2/1 -> AND2/2, AND/2
  NOT1/1 -> AND1/2, AND/1
  NOT/1 -> AND2/1, AND1/1
  AND2/1 -> OR/2
  AND/1 -> OR/1
  OR/1 -> OR1/1
  AND1/1 -> OR1/2
  OR1/1 -> Sum/1
  AND3/1 -> OR2/1
  AND4/1 -> OR2/2
  AND5/1 -> OR3/1
  OR2/1 -> OR3/2
  OR3/1 -> Carry/1

== system Approx_Multiplier_M2_AMA2_NAB12/AMA2_32 ==
  A : Inport
  B : Inport  Port=2
  Cin : Inport  Port=3
  AND{,1..5} (6 alike) : Logic  IconShape=distinctive  AllPortsSameDT=off  OutDataTypeStr=boolean
  NOT : Logic  Operator=NOT  IconShape=distinctive  AllPortsSameDT=off  OutDataTypeStr=boolean
  NOT1 : Logic  Operator=NOT  IconShape=distinctive  AllPortsSameDT=off  OutDataTypeStr=boolean
  NOT2 : Logic  Operator=NOT  IconShape=distinctive  AllPortsSameDT=off  OutDataTypeStr=boolean
  OR{,1..3} (4 alike) : Logic  Operator=OR  IconShape=distinctive  AllPortsSameDT=off  OutDataTypeStr=boolean
  Sum : Outport
  Carry : Outport  Port=2
  wires:
  A/1 -> AND4/1, AND5/1, NOT/1
  B/1 -> AND4/2, AND3/2, NOT1/1
  Cin/1 -> AND5/2, AND3/1, NOT2/1
  NOT2/1 -> AND2/2, AND/2
  NOT1/1 -> AND1/2, AND/1
  NOT/1 -> AND2/1, AND1/1
  AND2/1 -> OR/2
  AND/1 -> OR/1
  OR/1 -> OR1/1
  AND1/1 -> OR1/2
  OR1/1 -> Sum/1
  AND3/1 -> OR2/1
  AND4/1 -> OR2/2
  AND5/1 -> OR3/1
  OR2/1 -> OR3/2
  OR3/1 -> Carry/1

== system Approx_Multiplier_M2_AMA2_NAB12/AMA2_33 ==
  A : Inport
  B : Inport  Port=2
  Cin : Inport  Port=3
  AND{,1..5} (6 alike) : Logic  IconShape=distinctive  AllPortsSameDT=off  OutDataTypeStr=boolean
  NOT : Logic  Operator=NOT  IconShape=distinctive  AllPortsSameDT=off  OutDataTypeStr=boolean
  NOT1 : Logic  Operator=NOT  IconShape=distinctive  AllPortsSameDT=off  OutDataTypeStr=boolean
  NOT2 : Logic  Operator=NOT  IconShape=distinctive  AllPortsSameDT=off  OutDataTypeStr=boolean
  OR{,1..3} (4 alike) : Logic  Operator=OR  IconShape=distinctive  AllPortsSameDT=off  OutDataTypeStr=boolean
  Sum : Outport
  Carry : Outport  Port=2
  wires:
  A/1 -> AND4/1, AND5/1, NOT/1
  B/1 -> AND4/2, AND3/2, NOT1/1
  Cin/1 -> AND5/2, AND3/1, NOT2/1
  NOT2/1 -> AND2/2, AND/2
  NOT1/1 -> AND1/2, AND/1
  NOT/1 -> AND2/1, AND1/1
  AND2/1 -> OR/2
  AND/1 -> OR/1
  OR/1 -> OR1/1
  AND1/1 -> OR1/2
  OR1/1 -> Sum/1
  AND3/1 -> OR2/1
  AND4/1 -> OR2/2
  AND5/1 -> OR3/1
  OR2/1 -> OR3/2
  OR3/1 -> Carry/1

== system Approx_Multiplier_M2_AMA2_NAB12/AMA2_34 ==
  A : Inport
  B : Inport  Port=2
  Cin : Inport  Port=3
  AND{,1..5} (6 alike) : Logic  IconShape=distinctive  AllPortsSameDT=off  OutDataTypeStr=boolean
  NOT : Logic  Operator=NOT  IconShape=distinctive  AllPortsSameDT=off  OutDataTypeStr=boolean
  NOT1 : Logic  Operator=NOT  IconShape=distinctive  AllPortsSameDT=off  OutDataTypeStr=boolean
  NOT2 : Logic  Operator=NOT  IconShape=distinctive  AllPortsSameDT=off  OutDataTypeStr=boolean
  OR{,1..3} (4 alike) : Logic  Operator=OR  IconShape=distinctive  AllPortsSameDT=off  OutDataTypeStr=boolean
  Sum : Outport
  Carry : Outport  Port=2
  wires:
  A/1 -> AND4/1, AND5/1, NOT/1
  B/1 -> AND4/2, AND3/2, NOT1/1
  Cin/1 -> AND5/2, AND3/1, NOT2/1
  NOT2/1 -> AND2/2, AND/2
  NOT1/1 -> AND1/2, AND/1
  NOT/1 -> AND2/1, AND1/1
  AND2/1 -> OR/2
  AND/1 -> OR/1
  OR/1 -> OR1/1
  AND1/1 -> OR1/2
  OR1/1 -> Sum/1
  AND3/1 -> OR2/1
  AND4/1 -> OR2/2
  AND5/1 -> OR3/1
  OR2/1 -> OR3/2
  OR3/1 -> Carry/1

== system Approx_Multiplier_M2_AMA2_NAB12/AMA2_35 ==
  A : Inport
  B : Inport  Port=2
  Cin : Inport  Port=3
  AND{,1..5} (6 alike) : Logic  IconShape=distinctive  AllPortsSameDT=off  OutDataTypeStr=boolean
  NOT : Logic  Operator=NOT  IconShape=distinctive  AllPortsSameDT=off  OutDataTypeStr=boolean
  NOT1 : Logic  Operator=NOT  IconShape=distinctive  AllPortsSameDT=off  OutDataTypeStr=boolean
  NOT2 : Logic  Operator=NOT  IconShape=distinctive  AllPortsSameDT=off  OutDataTypeStr=boolean
  OR{,1..3} (4 alike) : Logic  Operator=OR  IconShape=distinctive  AllPortsSameDT=off  OutDataTypeStr=boolean
  Sum : Outport
  Carry : Outport  Port=2
  wires:
  A/1 -> AND4/1, AND5/1, NOT/1
  B/1 -> AND4/2, AND3/2, NOT1/1
  Cin/1 -> AND5/2, AND3/1, NOT2/1
  NOT2/1 -> AND2/2, AND/2
  NOT1/1 -> AND1/2, AND/1
  NOT/1 -> AND2/1, AND1/1
  AND2/1 -> OR/2
  AND/1 -> OR/1
  OR/1 -> OR1/1
  AND1/1 -> OR1/2
  OR1/1 -> Sum/1
  AND3/1 -> OR2/1
  AND4/1 -> OR2/2
  AND5/1 -> OR3/1
  OR2/1 -> OR3/2
  OR3/1 -> Carry/1

== system Approx_Multiplier_M2_AMA2_NAB12/AMA2_36 ==
  A : Inport
  B : Inport  Port=2
  Cin : Inport  Port=3
  AND{,1..5} (6 alike) : Logic  IconShape=distinctive  AllPortsSameDT=off  OutDataTypeStr=boolean
  NOT : Logic  Operator=NOT  IconShape=distinctive  AllPortsSameDT=off  OutDataTypeStr=boolean
  NOT1 : Logic  Operator=NOT  IconShape=distinctive  AllPortsSameDT=off  OutDataTypeStr=boolean
  NOT2 : Logic  Operator=NOT  IconShape=distinctive  AllPortsSameDT=off  OutDataTypeStr=boolean
  OR{,1..3} (4 alike) : Logic  Operator=OR  IconShape=distinctive  AllPortsSameDT=off  OutDataTypeStr=boolean
  Sum : Outport
  Carry : Outport  Port=2
  wires:
  A/1 -> AND4/1, AND5/1, NOT/1
  B/1 -> AND4/2, AND3/2, NOT1/1
  Cin/1 -> AND5/2, AND3/1, NOT2/1
  NOT2/1 -> AND2/2, AND/2
  NOT1/1 -> AND1/2, AND/1
  NOT/1 -> AND2/1, AND1/1
  AND2/1 -> OR/2
  AND/1 -> OR/1
  OR/1 -> OR1/1
  AND1/1 -> OR1/2
  OR1/1 -> Sum/1
  AND3/1 -> OR2/1
  AND4/1 -> OR2/2
  AND5/1 -> OR3/1
  OR2/1 -> OR3/2
  OR3/1 -> Carry/1

== system Approx_Multiplier_M2_AMA2_NAB12/AMA2_37 ==
  A : Inport
  B : Inport  Port=2
  Cin : Inport  Port=3
  AND{,1..5} (6 alike) : Logic  IconShape=distinctive  AllPortsSameDT=off  OutDataTypeStr=boolean
  NOT : Logic  Operator=NOT  IconShape=distinctive  AllPortsSameDT=off  OutDataTypeStr=boolean
  NOT1 : Logic  Operator=NOT  IconShape=distinctive  AllPortsSameDT=off  OutDataTypeStr=boolean
  NOT2 : Logic  Operator=NOT  IconShape=distinctive  AllPortsSameDT=off  OutDataTypeStr=boolean
  OR{,1..3} (4 alike) : Logic  Operator=OR  IconShape=distinctive  AllPortsSameDT=off  OutDataTypeStr=boolean
  Sum : Outport
  Carry : Outport  Port=2
  wires:
  A/1 -> AND4/1, AND5/1, NOT/1
  B/1 -> AND4/2, AND3/2, NOT1/1
  Cin/1 -> AND5/2, AND3/1, NOT2/1
  NOT2/1 -> AND2/2, AND/2
  NOT1/1 -> AND1/2, AND/1
  NOT/1 -> AND2/1, AND1/1
  AND2/1 -> OR/2
  AND/1 -> OR/1
  OR/1 -> OR1/1
  AND1/1 -> OR1/2
  OR1/1 -> Sum/1
  AND3/1 -> OR2/1
  AND4/1 -> OR2/2
  AND5/1 -> OR3/1
  OR2/1 -> OR3/2
  OR3/1 -> Carry/1

== system Approx_Multiplier_M2_AMA2_NAB12/AMA2_38 ==
  A : Inport
  B : Inport  Port=2
  Cin : Inport  Port=3
  AND{,1..5} (6 alike) : Logic  IconShape=distinctive  AllPortsSameDT=off  OutDataTypeStr=boolean
  NOT : Logic  Operator=NOT  IconShape=distinctive  AllPortsSameDT=off  OutDataTypeStr=boolean
  NOT1 : Logic  Operator=NOT  IconShape=distinctive  AllPortsSameDT=off  OutDataTypeStr=boolean
  NOT2 : Logic  Operator=NOT  IconShape=distinctive  AllPortsSameDT=off  OutDataTypeStr=boolean
  OR{,1..3} (4 alike) : Logic  Operator=OR  IconShape=distinctive  AllPortsSameDT=off  OutDataTypeStr=boolean
  Sum : Outport
  Carry : Outport  Port=2
  wires:
  A/1 -> AND4/1, AND5/1, NOT/1
  B/1 -> AND4/2, AND3/2, NOT1/1
  Cin/1 -> AND5/2, AND3/1, NOT2/1
  NOT2/1 -> AND2/2, AND/2
  NOT1/1 -> AND1/2, AND/1
  NOT/1 -> AND2/1, AND1/1
  AND2/1 -> OR/2
  AND/1 -> OR/1
  OR/1 -> OR1/1
  AND1/1 -> OR1/2
  OR1/1 -> Sum/1
  AND3/1 -> OR2/1
  AND4/1 -> OR2/2
  AND5/1 -> OR3/1
  OR2/1 -> OR3/2
  OR3/1 -> Carry/1
